simulink model "pisfuntestslx1"  (R2014a)
settings: Solver=ode45  StartTime=0.0  StopTime=10.0  FixedStep=0.14  RelTol=1e-3
libraries: powerlib x1
settings Model: Creator=Think127  LastModifiedBy=Think127

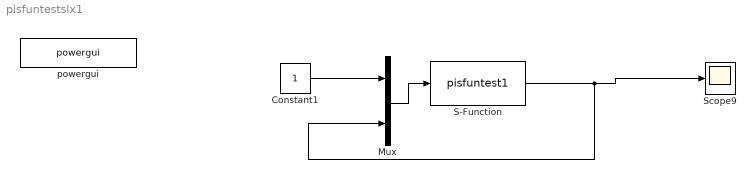
== system pisfuntestslx1 ==
  Constant1 : Constant
  Mux : Mux  Inputs=2
  S-Function : S-Function  FunctionName=pisfuntest1  EnableBusSupport=off
  Scope9 : Scope
      settings: TimeRange=2  YMin=39  YMax=41.5  SaveName=ScopeData4
  powergui : powerlib/powergui  Priority=1  SimulationMode=Discrete  SolverType=Tustin  SampleTime=1  frequency=60  SPID=off  DisableSnubberDevices=off  DisableRonSwitches=off  DisableVfSwitches=off  SwTol=0  Interpol=off  DisplayEquations=off  Ts=0  methode=off  frequencyindice=0  Pbase=100e6  ErrMax=1e-4  Iterations=50  UnitsV=kV  UnitsW=MW  FunctionMessages=off  echomessages=off  HookPort=off  EnableUseOfTLC=off  x0status=blocks  RestoreLinks=warning  ResistiveCurrentMeasurement=off  Frange=[0:2:500]  Ylog=off  Xlog=on  ShowGrid=off  save=off  variable=ZData  structure=0  ZoomFFT=on  StartTime=0.0  cycles=1  DisplayStyle=1  fundamental=60  FreqAxis=off  MaxFrequency=1000  frequencyindicesteady=1  RmsSteady=1  display=off
  wires:
  S-Function/1 -> Mux/2, Scope9/1
  Constant1/1 -> Mux/1
  Mux/1 -> S-Function/1
